simulink model "SCBattery_fuzzy"  (R2025b)
settings: Solver=ode15s  StartTime=20  StopTime=25  MaxStep=1e-4  MinStep=1e-6  RelTol=1e-3
undefined symbols (not defined in the file or in its folder): Ion, Lithium
libraries: spsCurrentMeasurementLib x4, spsMosfetLib x4, slpidlib x3, spsSeriesRLCBranchLib x3, spsVoltageMeasurementLib x3, spsBatteryLib x2, spsDiodeLib x2, spsDCVoltageSourceLib x2, simulink x2, autolibshared x1, fuzblock x1, spsSupercapacitorLib x1
settings Model: Creator=ankit  LastModifiedBy=44100
settings SolverCC: MaxOrder=3.0  ZeroCrossControl=DisableAll  ZeroCrossAlgorithm=Adaptive
settings DebuggingCC: IgnoredZcDiagnostic=none
settings RTWCC: GPUComputeCapability=3.5

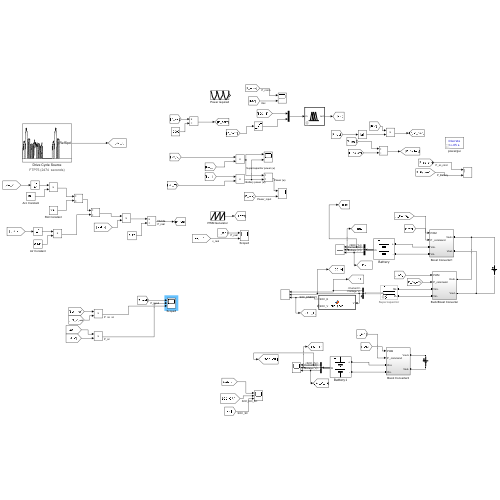
[thumbnail: Simulink's stored preview of the top-level diagram]
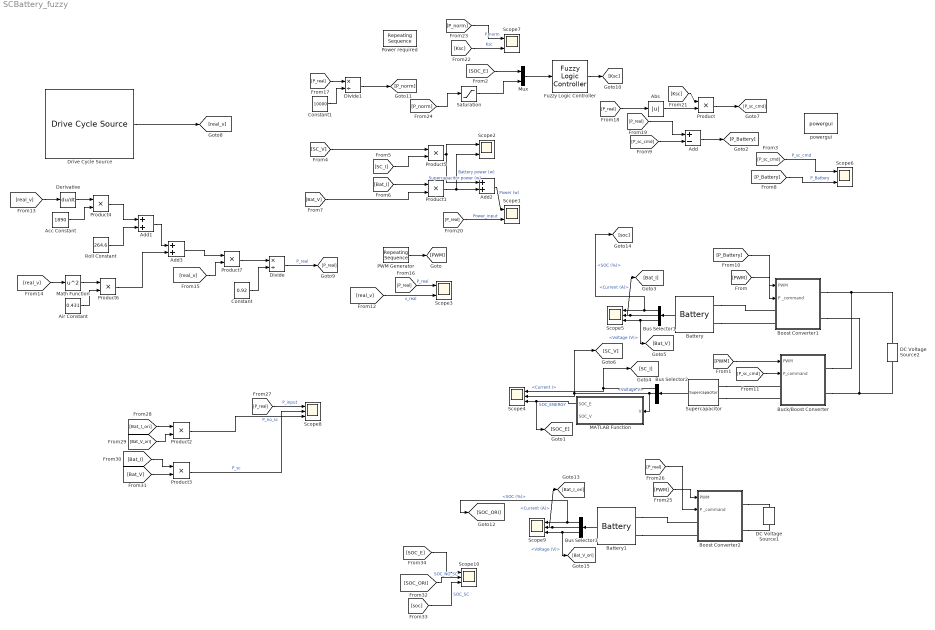
== system SCBattery_fuzzy ==
  Abs : Abs  SaturateOnIntegerOverflow=off
  Acc Constant : Constant  Value=1890
  Add : Sum  Inputs=+-
  Add1 : Sum
  Add2 : Sum
  Add3 : Sum
  Air Constant : Constant  Value=0.431
  Battery : spsBatteryLib/Battery  BatType=Lithium-Ion  NomV=42  NomQ=500  SOC=95  Batt_Tr=1  PresetModel=on  MaxQ=500  MinV=31.5  FullV=48.8875  Dis_rate=217.3913  R=0.00084  Normal_OP=452.1739  expZone="[45.3762      24.5652]"
      settings: LibrarySourceBlock=electricdrivelib/Extra Sources/Battery
  Battery1 : spsBatteryLib/Battery  BatType=Lithium-Ion  NomV=42  NomQ=500  SOC=95  Batt_Tr=1  PresetModel=on  MaxQ=500  MinV=31.5  FullV=48.8875  Dis_rate=217.3913  R=0.00084  Normal_OP=452.1739  expZone="[45.3762      24.5652]"
      settings: LibrarySourceBlock=electricdrivelib/Extra Sources/Battery
  Boost Converter1 : Subsystem
  Boost Converter2 : Subsystem
  Buck/Boost Converter : Subsystem
  Bus Selector1 : BusSelector  OutputSignals=SOC (%),Current (A),Voltage (V)
  Bus Selector2 : BusSelector  OutputSignals=Current I,Voltage V,SOC %
  Bus Selector3 : BusSelector  OutputSignals=SOC (%),Current (A),Voltage (V)
  Constant : Constant  Value=0.92
  Constant1 : Constant  Value=10000
  DC Voltage Source1 : spsDCVoltageSourceLib/DC Voltage Source  Amplitude=50  Measurements=Voltage
  DC Voltage Source2 : spsDCVoltageSourceLib/DC Voltage Source  Amplitude=50  Measurements=Voltage
  Derivative : Derivative
  Divide : Product  Inputs=*/
  Divide1 : Product  Inputs=*/
  Drive Cycle Source : autolibshared/Drive Cycle Source  cycleVar=FTP75  fileVar=cycleFTP75.mat  tfinal="2474  seconds"  cycleRepeat=off  outAccPort=off  outGearPort=off  gearList=No gear data  t_wot1=5  xdot_woto=0  xdot_wot1=30  t_wot2=20  xdot_wot2=0  t_wotend=30  srcUnit=m/s  outUnit=m/s  srcAccUnit=m/s/s  outAccUnit=m/s^2  dt=0  aMode=1  faultOption=off  velBnd=2  velBndUnit=mph  inUnit=m/s  timeBnd=1  failOption=off  stopSim=off  maxFaultCnt=10  maxFaultTime=2  maxTotFaultTime=15  traceOption=off  dtTrace=1  traceWindow=10  lastDCname=FTP75  lastOutUnit=mph  lastDT=0  lastTB=1  lastSB=2  forceCalcBound=off
  Fuzzy Logic Controller : fuzblock/Fuzzy Logic  Controller  FIS='sc_ems_regen.fis'  OutputSampleNumber=101  DataType=double  UseLookupTable=off  NumBreakpoints=10  FuzzifiedInputs=off  RuleFiringStrengths=off  RuleOutputs=off  AggregatedOutputs=off  SimulateUsing=Interpreted execution  OutOfRangeInputValueMessage=warning  NoRuleFiredMessage=warning  EmptyOutputFuzzySetMessage=warning
  MATLAB Function : MATLAB Function  TreatAsAtomicUnit=on
  Math Function : Math  Operator=square
  Mux : Mux  Inputs=2
  PWM Generator : simulink/Sources/Repeating Sequence  rep_seq_t=[0 0.0001]  rep_seq_y=[0 1]
  Power required : simulink/Sources/Repeating Sequence  rep_seq_t=[0 1 2 3 4 5 6 7 8 9 10]  rep_seq_y=[2000 1900 1700 1500 1400 1300 1300 1400 1500 1600 1700]
  Product{,2..4,6..7} (6 alike) : Product
  Product1 : Product  RndMeth=Zero
  Product5 : Product  RndMeth=Zero
  Roll Constant : Constant  Value=264.6
  Saturation : Saturate  UpperLimit=3  LowerLimit=-3
  Scope{1..3,6..7} (5 alike) : Scope  NumInputPorts=2
      Scope1 settings: ActiveDisplayYMinimum=-2299.9279428388272  ActiveDisplayYMaximum=20699.35148554945  DataLoggingSaveFormat=Array
      Scope2 settings: ActiveDisplayYMinimum=-2282.651401876873  ActiveDisplayYMaximum=20543.86261689186  DataLoggingVariableName=ScopeData3  DataLoggingSaveFormat=Array
      Scope3 settings: ActiveDisplayYMinimum=-1497.4446505772523  ActiveDisplayYMaximum=13477.001855195273  DataLoggingVariableName=ScopeData5  DataLoggingSaveFormat=Array
      Scope6 settings: ActiveDisplayYMinimum=-2284.340443196766  ActiveDisplayYMaximum=20559.063988770897  DataLoggingVariableName=ScopeData6  DataLoggingSaveFormat=Array
      Scope7 settings: ActiveDisplayYMinimum=-0.44306525201230423  ActiveDisplayYMaximum=0.095728009958294835  DataLoggingVariableName=ScopeData8  DataLoggingSaveFormat=Array
  Scope{4..5,8..10} (5 alike) : Scope  NumInputPorts=3
      Scope10 settings: ActiveDisplayYMinimum=95.120757001325543  ActiveDisplayYMaximum=95.167723352236536  DataLoggingVariableName=ScopeData10  DataLoggingSaveFormat=Array
      Scope4 settings: ActiveDisplayYMinimum=-18.227614227512753  ActiveDisplayYMaximum=26.129550693272527  DataLoggingVariableName=ScopeData4  DataLoggingSaveFormat=Array
      Scope5 settings: ActiveDisplayYMinimum=-50.612057754599583  ActiveDisplayYMaximum=455.5085197913964  DataLoggingSaveFormat=Array
      Scope8 settings: ActiveDisplayString=3  ActiveDisplayYMinimum=-2298.0492909344812  ActiveDisplayYMaximum=20682.315210592271  DataLoggingVariableName=ScopeData7  DataLoggingSaveFormat=Array
      Scope9 settings: ActiveDisplayYMinimum=-11.072505755634342  ActiveDisplayYMaximum=99.649741574628365  DataLoggingVariableName=ScopeData9  DataLoggingSaveFormat=Array
  Supercapacitor : spsSupercapacitorLib/Supercapacitor  C=10  Rdc=4e-3  Voltage=2.7  Ns=24  Np=1  Vinit=30  Temp=25  Nc=1  r=1e-9  epsilon=6.0208e-10  Ioc=10  Vself="[48  47.8  47.06  44.65]"
      settings: LibrarySourceBlock=electricdrivelib/Extra Sources/Supercapacitor
  powergui : spspowerguiLib/powergui  Priority=1  SimulationMode=Discrete  SampleTime=10e-6  frequency=60  Iterations=50  frequencyindice=0  Pbase=100e6  ErrMax=1e-4  UnitsV=kV  UnitsW=MW  buscounter=0  FunctionMessages=off  echomessages=off  EnableUseOfTLC=off  CurrentSourceSwitches=off  DisableSnubberDevices=off  DisableRonSwitches=off  DisableVfSwitches=off  DisplayEquations=off  AutomaticDiscreteSolvers=off  SolverType=Tustin/Backward Euler (TBE)  Interpol=off  ExternalGateDelay=off  methode=off  Ts=0  x0status=blocks  SPID=off  SwTol=0  HookPort=off  NonlinearTolerance=1e-4  nMaxIteration=100  ContinueOnMaxIteration=off  RestoreLinks=warning  ResistiveCurrentMeasurement=off  Frange=[0:1:1000]  Ylog=on  Xlog=on  ShowGrid=on  save=on  variable=ZDa  structure=donnee  ZoomFFT=off  StartTime=0.0  cycles=1  DisplayStyle=1  fundamental=60  FreqAxis=off  MaxFrequency=1000  frequencyindicesteady=10  RmsSteady=1  display=off
  wires:
  Bus Selector2/2 -> [SC_V], Scope4/2, MATLAB Function/1(V)  "<Voltage V>"
  Bus Selector1/3 -> [Bat_V], Scope5/3  "<Voltage (V)>"
  PWM Generator/1 -> [PWM]
  Supercapacitor/1 -> Bus Selector2/1
  Product1/1 -> Add2/2, Scope2/2  "Battery power (w)"
  [SC_I] -> Product5/2
  Bus Selector2/1 -> [SC_I], Scope4/1  "<Current I>"
  Bus Selector1/1 -> [soc], Scope5/1  "<SOC (%)>"
  Battery/1 -> Bus Selector1/1
  Bus Selector1/2 -> [Bat_I], Scope5/2  "<Current (A)>"
  [PWM] -> Buck/Boost Converter/1("PWM ")
  Add2/1 -> Scope1/1  "Power (w)"
  [Bat_I] -> Product1/1
  Product5/1 -> Add2/1, Scope2/1  "Supercapacitor power (w)"
  MATLAB Function/1(SOC_E) -> [SOC_E], Scope4/3  "SOC_ENERGY"
  [SOC_E] -> Mux/1
  Mux/1 -> Fuzzy Logic Controller/1
  Saturation/1 -> Mux/2
  Product/1 -> [P_sc_cmd]
  [P_sc_cmd] -> Add/2
  [P_sc_cmd] -> Buck/Boost Converter/2(P_command)
  Math Function/1 -> Product6/1
  Air Constant/1 -> Product6/2
  Product7/1 -> Divide/1
  [real_v] -> Derivative/1
  Derivative/1 -> Product4/1
  Product6/1 -> Add3/2
  Add1/1 -> Add3/1
  Constant/1 -> Divide/2
  Roll Constant/1 -> Add1/2
  [real_v] -> Product7/2
  Acc Constant/1 -> Product4/2
  Product4/1 -> Add1/1
  Add3/1 -> Product7/1
  [real_v] -> Scope3/2  "v_real"
  [real_v] -> Math Function/1
  Drive Cycle Source/1 -> [real_v]
  [P_real] -> Scope3/1  "P_real"
  [P_real] -> Divide1/1
  [P_real] -> Abs/1
  [P_real] -> Add/1
  Constant1/1 -> Divide1/2
  [P_real] -> Scope1/2  "Power_input"
  [SC_V] -> Product5/1
  [Bat_V] -> Product1/2
  Divide/1 -> [P_real]  "P_real"
  Abs/1 -> Product/2
  [P_sc_cmd] -> Scope6/1  "P_sc_cmd"
  Add/1 -> [P_Battery]
  [P_Battery] -> Scope6/2  "P_Battery"
  Fuzzy Logic Controller/1 -> [Ksc]
  [Ksc] -> Product/1
  [PWM] -> Boost Converter1/1("PWM ")
  [P_Battery] -> Boost Converter1/2(P _command)
  Divide1/1 -> [P_norm]
  [Ksc] -> Scope7/2  "Ksc"
  [P_norm] -> Scope7/1  "P_norm"
  [P_norm] -> Saturation/1
  [P_real] -> Boost Converter2/2(P _command)
  Battery1/1 -> Bus Selector3/1
  Bus Selector3/3 -> [Bat_V_ori], Scope9/3  "<Voltage (V)>"
  [PWM] -> Boost Converter2/1("PWM ")
  Bus Selector3/1 -> [SOC_ORI], Scope9/1  "<SOC (%)>"
  Bus Selector3/2 -> [Bat_I_ori], Scope9/2  "<Current (A)>"
  [P_real] -> Scope8/1  "P_input"
  [Bat_I_ori] -> Product2/1
  [Bat_V_ori] -> Product2/2
  Product2/1 -> Scope8/3  "P_no_sc"
  [Bat_I] -> Product3/1
  [Bat_V] -> Product3/2
  Product3/1 -> Scope8/2  "P_sc"
  [SOC_E] -> Scope10/1
  [soc] -> Scope10/3  "SOC_SC"
  [SOC_ORI] -> Scope10/2  "SOC_NO_SC"
  connections:
  Buck/Boost Converter/RConn2 -- Boost Converter1/RConn2 -- DC Voltage Source2/LConn1
  Buck/Boost Converter/RConn1 -- DC Voltage Source2/RConn1 -- Boost Converter1/RConn1
  Supercapacitor/LConn1 -- Buck/Boost Converter/LConn1
  Supercapacitor/LConn2 -- Buck/Boost Converter/LConn2
  Battery/LConn1 -- Boost Converter1/LConn1
  Battery/LConn2 -- Boost Converter1/LConn2
  Boost Converter2/RConn2 -- DC Voltage Source1/LConn1
  Boost Converter2/RConn1 -- DC Voltage Source1/RConn1
  Battery1/LConn1 -- Boost Converter2/LConn1
  Battery1/LConn2 -- Boost Converter2/LConn2

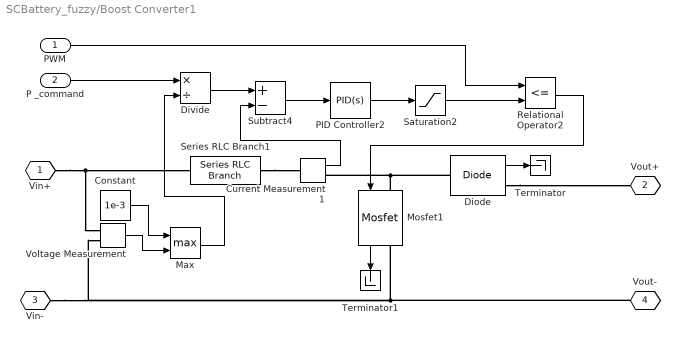
== system SCBattery_fuzzy/Boost Converter1 ==
  "PWM " : Inport
  P _command : Inport  Port=2
  Constant : Constant  Value=1e-3
  Current Measurement1 : spsCurrentMeasurementLib/Current Measurement  PhasorSimulation=off  OutputType=Complex  PSBequivalent=0
  Diode : spsDiodeLib/Diode  Ron=0.001  Lon=0  Vf=0.8  IC=0  UseSnubber=off  Rs=500  Cs=250e-9  Measurements=on
  Divide : Product  Inputs=*/
  Max : MinMax  Function=max  Inputs=2
  Mosfet1 : spsMosfetLib/Mosfet  Ron=0.1  Lon=0  Rd=0.01  Vfd=0  IC=0  Rs=1e5  Cs=inf  Measurements=on
  PID Controller2 : slpidlib/PID Controller  Controller=PID  Form=Parallel  TimeDomain=Continuous-time  UseExternalTs=off  SampleTime=-1  IntegratorMethod=Forward Euler  FilterMethod=Forward Euler  ControllerParametersSource=internal  P=1.5  I=0  UseKiTs=off  D=0  UseExternalDerivativeSource=off  N=100  UseFilter=on  TunerSelectOption=Transfer Function Based (PID Tuner App)  InitialConditionSource=internal  InitialConditionForIntegrator=0  InitialConditionForFilter=0  DifferentiatorICPrevScaledInput=0  ExternalReset=none  TrackingMode=off  Kt=1  LimitOutput=on  SatLimitsSource=internal  UpperSaturationLimit=0.9  LowerSaturationLimit=0  LinearizeAsGain=off  AntiWindupMode=back-calculation  Kb=1  LimitIntegrator=off  UpperIntegratorSaturationLimit=inf  LowerIntegratorSaturationLimit=-inf  POutMin=[]  POutMax=[]  IOutMin=[]  IOutMax=[]  DOutMin=[]  DOutMax=[]  NOutMin=[]  NOutMax=[]  SumOutMin=[]  SumOutMax=[]  SaturationOutMin=[]  SaturationOutMax=[]  PParamMin=[]  PParamMax=[]  IParamMin=[]  IParamMax=[]  DParamMin=[]  DParamMax=[]  NParamMin=[]  NParamMax=[]  KbParamMin=[]  KbParamMax=[]  KtParamMin=[]  KtParamMax=[]  KbOutMin=[]  KbOutMax=[]  KtOutMin=[]  KtOutMax=[]  IntegratorOutMin=[]  IntegratorOutMax=[]  FilterOutMin=[]  FilterOutMax=[]  SumI1OutMin=[]  SumI1OutMax=[]  SumI2OutMin=[]  SumI2OutMax=[]  SumI3OutMin=[]  SumI3OutMax=[]  SumI4OutMin=[]  SumI4OutMax=[]  SumDOutMin=[]  SumDOutMax=[]  DifferentiatorOutMin=[]  DifferentiatorOutMax=[]  FilterDiffOutCoefMin=[]  FilterDiffOutCoefMax=[]  ReciprocalOutMin=[]  ReciprocalOutMax=[]  SumDenOutMin=[]  SumDenOutMax=[]  SumNumOutMin=[]  SumNumOutMax=[]  DivideOutMin=[]  DivideOutMax=[]  UdiffTsProdOutMin=[]  UdiffTsProdOutMax=[]  NTsProdOutMin=[]  NTsProdOutMax=[]  UintegralTsProdOutMin=[]  UintegralTsProdOutMax=[]  UngainTsProdOutMin=[]  UngainTsProdOutMax=[]  ClampingZeroOutDataTypeStr=Inherit: Inherit via back propagation  ClampingZeroOutMin=[]  ClampingZeroOutMax=[]  FilterDenConstantOutDataTypeStr=Inherit: Inherit via back propagation  FilterDenConstantOutMin=[]  FilterDenConstantOutMax=[]  PCopyOutDataTypeStr=Inherit: Inherit via back propagation  PCopyOutMin=[]  PCopyOutMax=[]  NCopyOutDataTypeStr=Inherit: Inherit via back propagation  NCopyOutMin=[]  NCopyOutMax=[]  IntegratorContinuousStateAttributes=''  IntegratorStateMustResolveToSignalObject=off  IntegratorRTWStateStorageClass=Auto  FilterContinuousStateAttributes=''  FilterStateMustResolveToSignalObject=off  FilterRTWStateStorageClass=Auto  ParallelPVariant=InternalParameters  IdealPVariant=Disabled  IVariant=InternalParameters  DVariant=InternalParameters  IntegratorVariant=Continuous  SatVariant=Enabled  AWVariant=BackCalculation  PCopyVariant=Disabled  TRVariant=Disabled  FdbkBlocksVariant=Forward  IdealPFdbkVariant=Disabled  SatFdbkVariant=Disabled  DerivativeFilterVariant=ContFilter  NVariant=InternalParameters  NCopyVariant=Disabled  FilterICVariant=InternalICsFilter  IntegratorICVariant=InternalICs  ExternalResetVariant=Disabled  TRSumVariant=Passthrough  SumFdbkVariant=Disabled  SumVariant=Sum_PID  TsampFilterVariant=InternalTs  TsampNgainVariant=Passthrough  TsampIntegralVariant=Disabled_SignalSpec  ExternalSaturationOutDataTypeStr=Inherit: Same as second input  DerivativeSourceVariant=ErrorSignal  PreIntVariant=InternalPreInt
  Relational Operator2 : RelationalOperator  Operator=<=  OutDataTypeStr=boolean  InputSameDT=off
  Saturation2 : Saturate  UpperLimit=0.9  LowerLimit=0
  Series RLC Branch1 : spsSeriesRLCBranchLib/Series RLC Branch  LConnTagsString=__new0  RConnTagsString=__new0  BranchType=L  Resistance=1  Inductance=2e-3  SetiL0=off  InitialCurrent=0  Capacitance=1e-6  Setx0=off  InitialVoltage=0  Measurements=None
  Subtract4 : Sum  Inputs=+-
  Terminator : Terminator
  Terminator1 : Terminator
  Voltage Measurement : spsVoltageMeasurementLib/Voltage Measurement  PhasorSimulation=off  OutputType=Complex  PSBequivalent=0
  Vin+ : PMIOPort  Tag=PMCPort  Side=Left
  Vout+ : PMIOPort  Tag=PMCPort  Port=2  Side=Right
  Vin- : PMIOPort  Tag=PMCPort  Port=3  Side=Left
  Vout- : PMIOPort  Tag=PMCPort  Port=4  Side=Right
  wires:
  P _command/1 -> Divide/1
  Divide/1 -> Subtract4/1
  Current Measurement1/1 -> Subtract4/2
  "PWM "/1 -> Relational Operator2/1
  Subtract4/1 -> PID Controller2/1
  Diode/1 -> Terminator/1
  Mosfet1/1 -> Terminator1/1
  Relational Operator2/1 -> Mosfet1/1
  Voltage Measurement/1 -> Max/2
  Constant/1 -> Max/1
  Max/1 -> Divide/2
  PID Controller2/1 -> Saturation2/1
  Saturation2/1 -> Relational Operator2/2
  connections:
  Series RLC Branch1/RConn1 -- Current Measurement1/LConn1
  Vout-/RConn1 -- Voltage Measurement/LConn2 -- Vin-/RConn1 -- Mosfet1/RConn1
  Vin+/RConn1 -- Voltage Measurement/LConn1 -- Series RLC Branch1/LConn1
  Diode/LConn1 -- Mosfet1/LConn1 -- Current Measurement1/RConn1
  Diode/RConn1 -- Vout+/RConn1

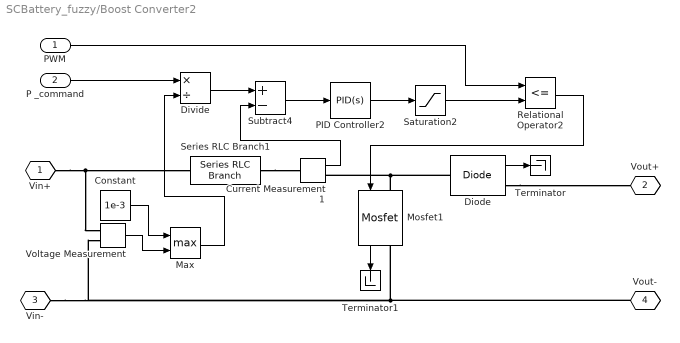
== system SCBattery_fuzzy/Boost Converter2 ==
  "PWM " : Inport
  P _command : Inport  Port=2
  Constant : Constant  Value=1e-3
  Current Measurement1 : spsCurrentMeasurementLib/Current Measurement  PhasorSimulation=off  OutputType=Complex  PSBequivalent=0
  Diode : spsDiodeLib/Diode  Ron=0.001  Lon=0  Vf=0.8  IC=0  UseSnubber=off  Rs=500  Cs=250e-9  Measurements=on
  Divide : Product  Inputs=*/
  Max : MinMax  Function=max  Inputs=2
  Mosfet1 : spsMosfetLib/Mosfet  Ron=0.1  Lon=0  Rd=0.01  Vfd=0  IC=0  Rs=1e5  Cs=inf  Measurements=on
  PID Controller2 : slpidlib/PID Controller  Controller=PID  Form=Parallel  TimeDomain=Continuous-time  UseExternalTs=off  SampleTime=-1  IntegratorMethod=Forward Euler  FilterMethod=Forward Euler  ControllerParametersSource=internal  P=1.5  I=0  UseKiTs=off  D=0  UseExternalDerivativeSource=off  N=100  UseFilter=on  TunerSelectOption=Transfer Function Based (PID Tuner App)  InitialConditionSource=internal  InitialConditionForIntegrator=0  InitialConditionForFilter=0  DifferentiatorICPrevScaledInput=0  ExternalReset=none  TrackingMode=off  Kt=1  LimitOutput=on  SatLimitsSource=internal  UpperSaturationLimit=0.9  LowerSaturationLimit=0  LinearizeAsGain=off  AntiWindupMode=back-calculation  Kb=1  LimitIntegrator=off  UpperIntegratorSaturationLimit=inf  LowerIntegratorSaturationLimit=-inf  POutMin=[]  POutMax=[]  IOutMin=[]  IOutMax=[]  DOutMin=[]  DOutMax=[]  NOutMin=[]  NOutMax=[]  SumOutMin=[]  SumOutMax=[]  SaturationOutMin=[]  SaturationOutMax=[]  PParamMin=[]  PParamMax=[]  IParamMin=[]  IParamMax=[]  DParamMin=[]  DParamMax=[]  NParamMin=[]  NParamMax=[]  KbParamMin=[]  KbParamMax=[]  KtParamMin=[]  KtParamMax=[]  KbOutMin=[]  KbOutMax=[]  KtOutMin=[]  KtOutMax=[]  IntegratorOutMin=[]  IntegratorOutMax=[]  FilterOutMin=[]  FilterOutMax=[]  SumI1OutMin=[]  SumI1OutMax=[]  SumI2OutMin=[]  SumI2OutMax=[]  SumI3OutMin=[]  SumI3OutMax=[]  SumI4OutMin=[]  SumI4OutMax=[]  SumDOutMin=[]  SumDOutMax=[]  DifferentiatorOutMin=[]  DifferentiatorOutMax=[]  FilterDiffOutCoefMin=[]  FilterDiffOutCoefMax=[]  ReciprocalOutMin=[]  ReciprocalOutMax=[]  SumDenOutMin=[]  SumDenOutMax=[]  SumNumOutMin=[]  SumNumOutMax=[]  DivideOutMin=[]  DivideOutMax=[]  UdiffTsProdOutMin=[]  UdiffTsProdOutMax=[]  NTsProdOutMin=[]  NTsProdOutMax=[]  UintegralTsProdOutMin=[]  UintegralTsProdOutMax=[]  UngainTsProdOutMin=[]  UngainTsProdOutMax=[]  ClampingZeroOutDataTypeStr=Inherit: Inherit via back propagation  ClampingZeroOutMin=[]  ClampingZeroOutMax=[]  FilterDenConstantOutDataTypeStr=Inherit: Inherit via back propagation  FilterDenConstantOutMin=[]  FilterDenConstantOutMax=[]  PCopyOutDataTypeStr=Inherit: Inherit via back propagation  PCopyOutMin=[]  PCopyOutMax=[]  NCopyOutDataTypeStr=Inherit: Inherit via back propagation  NCopyOutMin=[]  NCopyOutMax=[]  IntegratorContinuousStateAttributes=''  IntegratorStateMustResolveToSignalObject=off  IntegratorRTWStateStorageClass=Auto  FilterContinuousStateAttributes=''  FilterStateMustResolveToSignalObject=off  FilterRTWStateStorageClass=Auto  ParallelPVariant=InternalParameters  IdealPVariant=Disabled  IVariant=InternalParameters  DVariant=InternalParameters  IntegratorVariant=Continuous  SatVariant=Enabled  AWVariant=BackCalculation  PCopyVariant=Disabled  TRVariant=Disabled  FdbkBlocksVariant=Forward  IdealPFdbkVariant=Disabled  SatFdbkVariant=Disabled  DerivativeFilterVariant=ContFilter  NVariant=InternalParameters  NCopyVariant=Disabled  FilterICVariant=InternalICsFilter  IntegratorICVariant=InternalICs  ExternalResetVariant=Disabled  TRSumVariant=Passthrough  SumFdbkVariant=Disabled  SumVariant=Sum_PID  TsampFilterVariant=InternalTs  TsampNgainVariant=Passthrough  TsampIntegralVariant=Disabled_SignalSpec  ExternalSaturationOutDataTypeStr=Inherit: Same as second input  DerivativeSourceVariant=ErrorSignal  PreIntVariant=InternalPreInt
  Relational Operator2 : RelationalOperator  Operator=<=  OutDataTypeStr=boolean  InputSameDT=off
  Saturation2 : Saturate  UpperLimit=0.9  LowerLimit=0
  Series RLC Branch1 : spsSeriesRLCBranchLib/Series RLC Branch  LConnTagsString=__new0  RConnTagsString=__new0  BranchType=L  Resistance=1  Inductance=2e-3  SetiL0=off  InitialCurrent=0  Capacitance=1e-6  Setx0=off  InitialVoltage=0  Measurements=None
  Subtract4 : Sum  Inputs=+-
  Terminator : Terminator
  Terminator1 : Terminator
  Voltage Measurement : spsVoltageMeasurementLib/Voltage Measurement  PhasorSimulation=off  OutputType=Complex  PSBequivalent=0
  Vin+ : PMIOPort  Tag=PMCPort  Side=Left
  Vout+ : PMIOPort  Tag=PMCPort  Port=2  Side=Right
  Vin- : PMIOPort  Tag=PMCPort  Port=3  Side=Left
  Vout- : PMIOPort  Tag=PMCPort  Port=4  Side=Right
  wires:
  P _command/1 -> Divide/1
  Divide/1 -> Subtract4/1
  Current Measurement1/1 -> Subtract4/2
  "PWM "/1 -> Relational Operator2/1
  Subtract4/1 -> PID Controller2/1
  Diode/1 -> Terminator/1
  Mosfet1/1 -> Terminator1/1
  Relational Operator2/1 -> Mosfet1/1
  Voltage Measurement/1 -> Max/2
  Constant/1 -> Max/1
  Max/1 -> Divide/2
  PID Controller2/1 -> Saturation2/1
  Saturation2/1 -> Relational Operator2/2
  connections:
  Series RLC Branch1/RConn1 -- Current Measurement1/LConn1
  Vout-/RConn1 -- Voltage Measurement/LConn2 -- Vin-/RConn1 -- Mosfet1/RConn1
  Vin+/RConn1 -- Voltage Measurement/LConn1 -- Series RLC Branch1/LConn1
  Diode/LConn1 -- Mosfet1/LConn1 -- Current Measurement1/RConn1
  Diode/RConn1 -- Vout+/RConn1

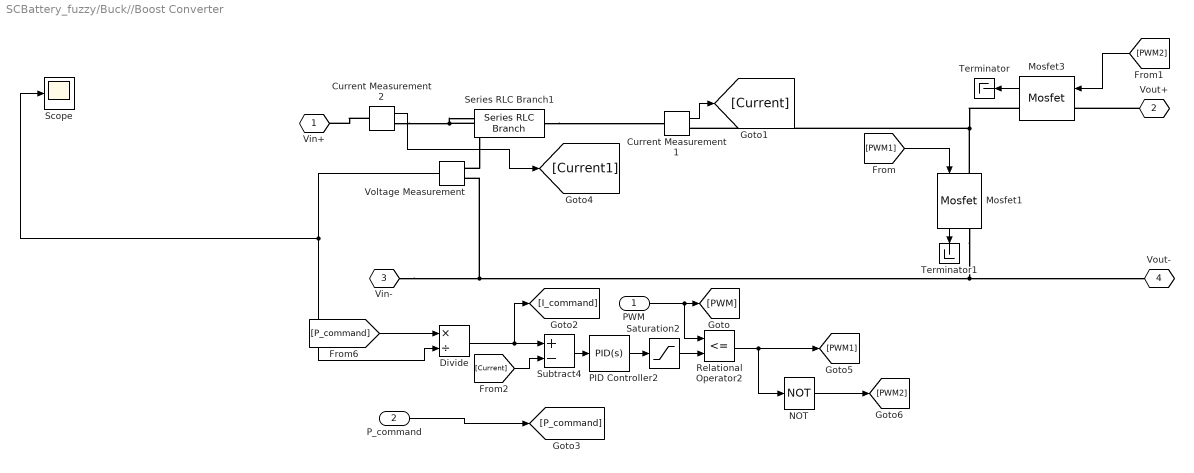
== system SCBattery_fuzzy/Buck//Boost Converter ==
  "PWM " : Inport
  P_command : Inport  Port=2
  Current Measurement1 : spsCurrentMeasurementLib/Current Measurement  PhasorSimulation=off  OutputType=Complex  PSBequivalent=0
  Current Measurement2 : spsCurrentMeasurementLib/Current Measurement  PhasorSimulation=off  OutputType=Complex  PSBequivalent=0
  Divide : Product  Inputs=*/
  Mosfet1 : spsMosfetLib/Mosfet  Ron=0.1  Lon=0  Rd=0.01  Vfd=0  IC=0  Rs=1e5  Cs=inf  Measurements=on
  Mosfet3 : spsMosfetLib/Mosfet  Ron=0.1  Lon=0  Rd=0.01  Vfd=0  IC=0  Rs=1e5  Cs=inf  Measurements=on
  NOT : Logic  Operator=NOT  IconShape=distinctive  AllPortsSameDT=off  OutDataTypeStr=boolean
  PID Controller2 : slpidlib/PID Controller  Controller=PID  Form=Parallel  TimeDomain=Continuous-time  UseExternalTs=off  SampleTime=-1  IntegratorMethod=Forward Euler  FilterMethod=Forward Euler  ControllerParametersSource=internal  P=1.5  I=1  UseKiTs=off  D=0  UseExternalDerivativeSource=off  N=100  UseFilter=on  TunerSelectOption=Transfer Function Based (PID Tuner App)  InitialConditionSource=internal  InitialConditionForIntegrator=0  InitialConditionForFilter=0  DifferentiatorICPrevScaledInput=0  ExternalReset=none  TrackingMode=off  Kt=1  LimitOutput=off  SatLimitsSource=internal  UpperSaturationLimit=inf  LowerSaturationLimit=-inf  LinearizeAsGain=off  AntiWindupMode=none  Kb=1  LimitIntegrator=off  UpperIntegratorSaturationLimit=inf  LowerIntegratorSaturationLimit=-inf  POutMin=[]  POutMax=[]  IOutMin=[]  IOutMax=[]  DOutMin=[]  DOutMax=[]  NOutMin=[]  NOutMax=[]  SumOutMin=[]  SumOutMax=[]  SaturationOutMin=[]  SaturationOutMax=[]  PParamMin=[]  PParamMax=[]  IParamMin=[]  IParamMax=[]  DParamMin=[]  DParamMax=[]  NParamMin=[]  NParamMax=[]  KbParamMin=[]  KbParamMax=[]  KtParamMin=[]  KtParamMax=[]  KbOutMin=[]  KbOutMax=[]  KtOutMin=[]  KtOutMax=[]  IntegratorOutMin=[]  IntegratorOutMax=[]  FilterOutMin=[]  FilterOutMax=[]  SumI1OutMin=[]  SumI1OutMax=[]  SumI2OutMin=[]  SumI2OutMax=[]  SumI3OutMin=[]  SumI3OutMax=[]  SumI4OutMin=[]  SumI4OutMax=[]  SumDOutMin=[]  SumDOutMax=[]  DifferentiatorOutMin=[]  DifferentiatorOutMax=[]  FilterDiffOutCoefMin=[]  FilterDiffOutCoefMax=[]  ReciprocalOutMin=[]  ReciprocalOutMax=[]  SumDenOutMin=[]  SumDenOutMax=[]  SumNumOutMin=[]  SumNumOutMax=[]  DivideOutMin=[]  DivideOutMax=[]  UdiffTsProdOutMin=[]  UdiffTsProdOutMax=[]  NTsProdOutMin=[]  NTsProdOutMax=[]  UintegralTsProdOutMin=[]  UintegralTsProdOutMax=[]  UngainTsProdOutMin=[]  UngainTsProdOutMax=[]  ClampingZeroOutDataTypeStr=Inherit: Inherit via back propagation  ClampingZeroOutMin=[]  ClampingZeroOutMax=[]  FilterDenConstantOutDataTypeStr=Inherit: Inherit via back propagation  FilterDenConstantOutMin=[]  FilterDenConstantOutMax=[]  PCopyOutDataTypeStr=Inherit: Inherit via back propagation  PCopyOutMin=[]  PCopyOutMax=[]  NCopyOutDataTypeStr=Inherit: Inherit via back propagation  NCopyOutMin=[]  NCopyOutMax=[]  IntegratorContinuousStateAttributes=''  IntegratorStateMustResolveToSignalObject=off  IntegratorRTWStateStorageClass=Auto  FilterContinuousStateAttributes=''  FilterStateMustResolveToSignalObject=off  FilterRTWStateStorageClass=Auto  ParallelPVariant=InternalParameters  IdealPVariant=Disabled  IVariant=InternalParameters  DVariant=InternalParameters  IntegratorVariant=Continuous  SatVariant=Disabled  AWVariant=Passthrough  PCopyVariant=Disabled  TRVariant=Disabled  FdbkBlocksVariant=Forward  IdealPFdbkVariant=Disabled  SatFdbkVariant=Disabled  DerivativeFilterVariant=ContFilter  NVariant=InternalParameters  NCopyVariant=Disabled  FilterICVariant=InternalICsFilter  IntegratorICVariant=InternalICs  ExternalResetVariant=Disabled  TRSumVariant=Passthrough  SumFdbkVariant=Disabled  SumVariant=Sum_PID  TsampFilterVariant=InternalTs  TsampNgainVariant=Passthrough  TsampIntegralVariant=Disabled_SignalSpec  ExternalSaturationOutDataTypeStr=Inherit: Same as second input  DerivativeSourceVariant=ErrorSignal  PreIntVariant=InternalPreInt
  Relational Operator2 : RelationalOperator  Operator=<=  OutDataTypeStr=boolean  InputSameDT=off
  Saturation2 : Saturate  UpperLimit=1  LowerLimit=0
  Scope : Scope
      settings: ActiveDisplayYMinimum=14.984365899203418  ActiveDisplayYMaximum=16.112848664230761  DataLoggingVariableName=ScopeData2
  Series RLC Branch1 : spsSeriesRLCBranchLib/Series RLC Branch  LConnTagsString=__new0  RConnTagsString=__new0  BranchType=L  Resistance=1  Inductance=7e-3  SetiL0=off  InitialCurrent=0  Capacitance=1e-6  Setx0=off  InitialVoltage=0  Measurements=None
  Subtract4 : Sum  Inputs=+-
  Terminator : Terminator
  Terminator1 : Terminator
  Voltage Measurement : spsVoltageMeasurementLib/Voltage Measurement  PhasorSimulation=off  OutputType=Complex  PSBequivalent=0
  Vin+ : PMIOPort  Tag=PMCPort  Side=Left
  Vout+ : PMIOPort  Tag=PMCPort  Port=2  Side=Right
  Vin- : PMIOPort  Tag=PMCPort  Port=3  Side=Left
  Vout- : PMIOPort  Tag=PMCPort  Port=4  Side=Right
  wires:
  Saturation2/1 -> Relational Operator2/2
  PID Controller2/1 -> Saturation2/1
  Subtract4/1 -> PID Controller2/1
  "PWM "/1 -> Relational Operator2/1, [PWM]
  Divide/1 -> [I_command], Subtract4/1
  [Current] -> Subtract4/2
  Current Measurement1/1 -> [Current]
  Mosfet3/1 -> Terminator/1
  Mosfet1/1 -> Terminator1/1
  Voltage Measurement/1 -> Scope/1, Divide/2
  P_command/1 -> [P_command]
  [P_command] -> Divide/1
  Current Measurement2/1 -> [Current1]
  Relational Operator2/1 -> NOT/1, [PWM1]
  NOT/1 -> [PWM2]
  [PWM1] -> Mosfet1/1
  [PWM2] -> Mosfet3/1
  connections:
  Vin-/RConn1 -- Voltage Measurement/LConn2 -- Vout-/RConn1 -- Mosfet1/RConn1
  Series RLC Branch1/LConn1 -- Voltage Measurement/LConn1 -- Current Measurement2/RConn1
  Mosfet1/LConn1 -- Mosfet3/RConn1 -- Current Measurement1/RConn1
  Series RLC Branch1/RConn1 -- Current Measurement1/LConn1
  Vout+/RConn1 -- Mosfet3/LConn1
  Current Measurement2/LConn1 -- Vin+/RConn1

== matlab function SCBattery_fuzzy/MATLAB Function ==
  data: V input; SOC_E output; SOC_V output
function [SOC_E, SOC_V] = SC_SOC(V)
% ============================================
%   Supercapacitor SOC Calculation
%   输出两个信号：
%   SOC_E —— 能量型 SOC（给模糊控制器）
%   SOC_V —— 电压型 SOC（给保护）
% ============================================

%% ===== 超级电容参数 =====
Vcell_rated = 2.7;      % 单颗额定电压
N_series    = 16;       
Vmax        = Vcell_rated * N_series;   % ≈ 43.2 V
Vmin        = 16;        % 你模型里的最低运行电压

%% ===== 电压型 SOC =====
SOC_V = (V - Vmin) / (Vmax - Vmin);
SOC_V = max(0, min(1, SOC_V));   % 限幅

%% ===== 能量型 SOC =====
SOC_E = (V.^2 - Vmin^2) / (Vmax^2 - Vmin^2);
SOC_E = max(0, min(1, SOC_E));   % 限幅

end
